simulink model "Combined_Experiment_Jan23_2020a"  (R2020a)
settings: Solver=FixedStepAuto  StartTime=0.0  StopTime=tsim  FixedStep=baseRate  RelTol=1e-3  EnableMultiTasking=on
undefined symbols (not defined in the file): b0, b1, b_out, baseRate, CHASER_ABSOLUTE_POSITION, DiscIntNeverNeededParam, drop_states_ARM, drop_states_BLACK, drop_states_BLUE, drop_states_RED, F_Black_X_nominal, F_Black_Y_nominal, F_Blue_X_nominal, F_Blue_Y_nominal, F_red_X_nominal, F_red_Y_nominal, F_thrusters_BLACK, F_thrusters_BLUE, F_thrusters_RED, Gamma1_el, Gamma1_sh, Gamma1_wr, Gamma2_el, Gamma2_sh, Gamma2_wr, Gamma3_el, Gamma3_sh, Gamma3_wr, Gamma4_el, Gamma4_sh, Gamma4_wr, Gamma5_el, Gamma5_sh, Gamma5_wr, Gamma6_el, Gamma6_sh, Gamma6_wr, home_states_BLACK, home_states_BLUE, home_states_RED, init_states_BLACK, init_states_BLUE, init_states_RED, Kd_tb, Kd_tblue, Kd_tr, Kd_xb, Kd_xblue, Kd_xr, Kd_yb, Kd_yblue, Kd_yr, Kp_tb, Kp_tblue, Kp_tr, Kp_xb, Kp_xblue, Kp_xr, Kp_yb, Kp_yblue ... (+31)
libraries: dspstat3 x18, raspberrypiBasiclib x10, dspsigops x9, embdlinuxlib x8, MainLibrary x8, simulink x7, mspfiltlib x3, dsparch4 x3, etargetslib x1, sensehatlib x1
(part 5 of 11)

== system Combined_Experiment_Jan23_2020a/Phase #3: Experiment/Change BLUE Behavior/Sub-Phase #3  ==
  note: Additional blocks are stored here.
  note: A simple PD control law is used here to command the platform to it's initial position, as defined in the initializer.
  note: Additional Blocks
  note: PD Control Law - BLUE
  Action Port : ActionPort  ActionPortLabel=elseif( u1 < u4)
  BLACK_Rz : DataStoreRead  DataStoreName=BLUE_Rz
  BLACK_RzD1 : Subsystem
  BLACK_Tz : DataStoreWrite  DataStoreName=BLUE_Tz
  BLUE_Fx : DataStoreWrite  DataStoreName=BLUE_Fx
  BLUE_Fy : DataStoreWrite  DataStoreName=BLUE_Fy
  BLUE_Px : DataStoreRead  DataStoreName=BLUE_Px
  "BLUE_Py " : DataStoreRead  DataStoreName=BLUE_Py
  Constant : Constant  Value=xLength/2
  Constant1 : Constant  Value=yLength/2
  Custom Discrete PD (Attitude) : Subsystem
  Custom Discrete PD (X-Position) : Subsystem
  Custom Discrete PD (Y-Position) : Subsystem
  Data Store Write1 : DataStoreWrite  DataStoreName=Float_State
  Hough Control : Subsystem
  Puck State : Constant
  Subtract : Sum  Inputs=+-
  Subtract1 : Sum  Inputs=+-
  wires:
  Puck State/1 -> Data Store Write1/1
  BLACK_RzD1/1(Ref) -> Hough Control/1(Ref)
  BLACK_Rz/1 -> Hough Control/2(Act)
  BLUE_Px/1 -> Subtract/2
  "BLUE_Py "/1 -> Subtract1/2
  Subtract1/1 -> Custom Discrete PD (Y-Position)/1(ey)
  Subtract/1 -> Custom Discrete PD (X-Position)/1(ex)
  Custom Discrete PD (Y-Position)/1(Fy) -> BLUE_Fy/1
  Hough Control/1(Err) -> Custom Discrete PD (Attitude)/1(ez)
  Custom Discrete PD (Attitude)/1(Tz) -> BLACK_Tz/1
  Custom Discrete PD (X-Position)/1(Fx) -> BLUE_Fx/1
  Constant1/1 -> Subtract1/1
  Constant/1 -> Subtract/1

== system Combined_Experiment_Jan23_2020a/Phase #3: Experiment/Change BLUE Behavior/Sub-Phase #4 ==
  note: Additional blocks are stored here.
  note: A simple PD control law is used here to command the platform to it's initial position, as defined in the initializer.
  note: Additional Blocks
  note: PD Control Law - BLUE
  Action Port : ActionPort  ActionPortLabel=elseif( u1 < u5)
  BLACK_Rz : DataStoreRead  DataStoreName=BLUE_Rz
  BLACK_RzD1 : Subsystem
  BLACK_Tz : DataStoreWrite  DataStoreName=BLUE_Tz
  BLUE_Fx : DataStoreWrite  DataStoreName=BLUE_Fx
  BLUE_Fy : DataStoreWrite  DataStoreName=BLUE_Fy
  BLUE_Px : DataStoreRead  DataStoreName=BLUE_Px
  "BLUE_Py " : DataStoreRead  DataStoreName=BLUE_Py
  Constant : Constant  Value=xLength/2
  Constant1 : Constant  Value=yLength/2
  Custom Discrete PD (Attitude) : Subsystem
  Custom Discrete PD (X-Position) : Subsystem
  Custom Discrete PD (Y-Position) : Subsystem
  Data Store Write1 : DataStoreWrite  DataStoreName=Float_State
  Hough Control : Subsystem
  Puck State : Constant
  Subtract : Sum  Inputs=+-
  Subtract1 : Sum  Inputs=+-
  wires:
  Puck State/1 -> Data Store Write1/1
  BLACK_RzD1/1(Ref) -> Hough Control/1(Ref)
  BLACK_Rz/1 -> Hough Control/2(Act)
  BLUE_Px/1 -> Subtract/2
  "BLUE_Py "/1 -> Subtract1/2
  Subtract1/1 -> Custom Discrete PD (Y-Position)/1(ey)
  Subtract/1 -> Custom Discrete PD (X-Position)/1(ex)
  Custom Discrete PD (Y-Position)/1(Fy) -> BLUE_Fy/1
  Hough Control/1(Err) -> Custom Discrete PD (Attitude)/1(ez)
  Custom Discrete PD (Attitude)/1(Tz) -> BLACK_Tz/1
  Custom Discrete PD (X-Position)/1(Fx) -> BLUE_Fx/1
  Constant1/1 -> Subtract1/1
  Constant/1 -> Subtract/1

== system Combined_Experiment_Jan23_2020a/Phase #3: Experiment/Change BLUE Behavior/Subsystem ==
  Universal_Time : DataStoreRead  DataStoreName=Univ_Time
  Time : Outport  VectorParamsAs1DForOutWhenUnconnected=off
  wires:
  Universal_Time/1 -> Time/1

== system Combined_Experiment_Jan23_2020a/Phase #3: Experiment/Change RED Behavior/Sub-Phase #1 ==
  note: Additional Blocks
  note: Additional blocks are stored above. Note that to control attitude using the RW, simply replace RED_Tz with RED_Tz_RW.
  note: Feedforward control
  note: ARM Control Law - RED
  Action Port : ActionPort  ActionPortLabel=if(u1 < u2)
  Constant1 : Constant  Value=0
  Constant4 : Constant  Value=platformSelection
  Data Store Write3 : DataStoreWrite  DataStoreName=Float_State
  Demux1 : Demux  Outputs=3
  If : If  IfExpression=u1 == 4 | u1 == 5 | u1 == 10 | u1 == 11
  Mux3 : Mux  Inputs=3
  Product : Product  Multiplication=Matrix(*)
  Puck State : Constant
  RED : Subsystem  TreatAsAtomicUnit=on
  RED+ARM : Subsystem  TreatAsAtomicUnit=on
  RED_Desired_Ax : DataStoreRead  DataStoreName=RED_Desired_Ax
  RED_Desired_Ay : DataStoreRead  DataStoreName=RED_Desired_Ay
  RED_Desired_Omega : DataStoreRead  DataStoreName=RED_Desired_Alpha
  RED_Fx : DataStoreWrite  DataStoreName=RED_Fx
  RED_Fy : DataStoreWrite  DataStoreName=RED_Fy
  RED_Tz : DataStoreWrite  DataStoreName=RED_Tz
  RED_Tz_RW : DataStoreWrite  DataStoreName=RED_Tz_RW
  calculate_mass_matrix : MATLAB Function  TreatAsAtomicUnit=on
  wires:
  Constant1/1 -> RED_Tz_RW/1
  Puck State/1 -> Data Store Write3/1
  Product/1 -> Demux1/1
  RED_Desired_Omega/1 -> Mux3/3
  RED_Desired_Ay/1 -> Mux3/2
  calculate_mass_matrix/1(M) -> Product/1
  RED_Desired_Ax/1 -> Mux3/1
  Mux3/1 -> Product/2
  Demux1/1 -> RED_Fx/1
  Demux1/2 -> RED_Fy/1
  Demux1/3 -> RED_Tz/1
  If/1 -> RED+ARM/Action
  If/2 -> RED/Action
  Constant4/1 -> If/1

== system Combined_Experiment_Jan23_2020a/Phase #3: Experiment/Change RED Behavior/Sub-Phase #2  ==
  note: Feedforward control
  note: Additional Blocks
  note: ARM Control Law - RED
  note: Additional blocks are stored above. Note that to control attitude using the RW, simply replace RED_Tz with RED_Tz_RW.
  Action Port : ActionPort  ActionPortLabel=elseif(u1 < u3)
  Constant1 : Constant  Value=0
  Constant4 : Constant  Value=platformSelection
  Data Store Write3 : DataStoreWrite  DataStoreName=Float_State
  Demux1 : Demux  Outputs=3
  If : If  IfExpression=u1 == 4 | u1 == 5 | u1 == 10 | u1 == 11
  Mux3 : Mux  Inputs=3
  Product : Product  Multiplication=Matrix(*)
  Puck State : Constant
  RED : Subsystem  TreatAsAtomicUnit=on
  RED+ARM : Subsystem  TreatAsAtomicUnit=on
  RED_Desired_Ax : DataStoreRead  DataStoreName=RED_Desired_Ax
  RED_Desired_Ay : DataStoreRead  DataStoreName=RED_Desired_Ay
  RED_Desired_Omega : DataStoreRead  DataStoreName=RED_Desired_Alpha
  RED_Fx : DataStoreWrite  DataStoreName=RED_Fx
  RED_Fy : DataStoreWrite  DataStoreName=RED_Fy
  RED_Tz : DataStoreWrite  DataStoreName=RED_Tz
  RED_Tz_RW : DataStoreWrite  DataStoreName=RED_Tz_RW
  calculate_mass_matrix : MATLAB Function  TreatAsAtomicUnit=on
  wires:
  Demux1/1 -> RED_Fx/1
  Mux3/1 -> Product/2
  Demux1/3 -> RED_Tz/1
  calculate_mass_matrix/1(M) -> Product/1
  Product/1 -> Demux1/1
  Demux1/2 -> RED_Fy/1
  Constant1/1 -> RED_Tz_RW/1
  RED_Desired_Omega/1 -> Mux3/3
  Puck State/1 -> Data Store Write3/1
  Constant4/1 -> If/1
  If/2 -> RED/Action
  RED_Desired_Ay/1 -> Mux3/2
  If/1 -> RED+ARM/Action
  RED_Desired_Ax/1 -> Mux3/1

== system Combined_Experiment_Jan23_2020a/Phase #3: Experiment/Change RED Behavior/Sub-Phase #3  ==
  note: Feedforward control
  note: Additional Blocks
  note: ARM Control Law - RED
  note: Additional blocks are stored above. Note that to control attitude using the RW, simply replace RED_Tz with RED_Tz_RW.
  Action Port : ActionPort  ActionPortLabel=elseif( u1 < u4)
  Constant1 : Constant  Value=0
  Constant4 : Constant  Value=platformSelection
  Data Store Write3 : DataStoreWrite  DataStoreName=Float_State
  Demux1 : Demux  Outputs=3
  If : If  IfExpression=u1 == 4 | u1 == 5 | u1 == 10 | u1 == 11
  Mux3 : Mux  Inputs=3
  Product : Product  Multiplication=Matrix(*)
  Puck State : Constant
  RED : Subsystem  TreatAsAtomicUnit=on
  RED+ARM : Subsystem  TreatAsAtomicUnit=on
  RED_Desired_Ax : DataStoreRead  DataStoreName=RED_Desired_Ax
  RED_Desired_Ay : DataStoreRead  DataStoreName=RED_Desired_Ay
  RED_Desired_Omega : DataStoreRead  DataStoreName=RED_Desired_Alpha
  RED_Fx : DataStoreWrite  DataStoreName=RED_Fx
  RED_Fy : DataStoreWrite  DataStoreName=RED_Fy
  RED_Tz : DataStoreWrite  DataStoreName=RED_Tz
  RED_Tz_RW : DataStoreWrite  DataStoreName=RED_Tz_RW
  calculate_mass_matrix : MATLAB Function  TreatAsAtomicUnit=on
  wires:
  Demux1/1 -> RED_Fx/1
  Mux3/1 -> Product/2
  calculate_mass_matrix/1(M) -> Product/1
  Product/1 -> Demux1/1
  Demux1/2 -> RED_Fy/1
  Constant1/1 -> RED_Tz_RW/1
  RED_Desired_Omega/1 -> Mux3/3
  Puck State/1 -> Data Store Write3/1
  Constant4/1 -> If/1
  If/2 -> RED/Action
  RED_Desired_Ay/1 -> Mux3/2
  If/1 -> RED+ARM/Action
  RED_Desired_Ax/1 -> Mux3/1
  Demux1/3 -> RED_Tz/1

== system Combined_Experiment_Jan23_2020a/Phase #3: Experiment/Change RED Behavior/Sub-Phase #4 ==
  note: Feedforward control
  note: Additional Blocks
  note: ARM Control Law - RED
  note: Additional blocks are stored above. Note that to control attitude using the RW, simply replace RED_Tz with RED_Tz_RW.
  Action Port : ActionPort  ActionPortLabel=elseif( u1 < u5)
  Constant1 : Constant  Value=0
  Constant4 : Constant  Value=platformSelection
  Data Store Write3 : DataStoreWrite  DataStoreName=Float_State
  Demux1 : Demux  Outputs=3
  If : If  IfExpression=u1 == 4 | u1 == 5 | u1 == 10 | u1 == 11
  Mux3 : Mux  Inputs=3
  Product : Product  Multiplication=Matrix(*)
  Puck State : Constant
  RED : Subsystem  TreatAsAtomicUnit=on
  RED+ARM : Subsystem  TreatAsAtomicUnit=on
  RED_Desired_Ax : DataStoreRead  DataStoreName=RED_Desired_Ax
  RED_Desired_Ay : DataStoreRead  DataStoreName=RED_Desired_Ay
  RED_Desired_Omega : DataStoreRead  DataStoreName=RED_Desired_Alpha
  RED_Fx : DataStoreWrite  DataStoreName=RED_Fx
  RED_Fy : DataStoreWrite  DataStoreName=RED_Fy
  RED_Tz : DataStoreWrite  DataStoreName=RED_Tz
  RED_Tz_RW : DataStoreWrite  DataStoreName=RED_Tz_RW
  calculate_mass_matrix : MATLAB Function  TreatAsAtomicUnit=on
  wires:
  Demux1/1 -> RED_Fx/1
  Mux3/1 -> Product/2
  Demux1/3 -> RED_Tz/1
  calculate_mass_matrix/1(M) -> Product/1
  Product/1 -> Demux1/1
  Demux1/2 -> RED_Fy/1
  Constant1/1 -> RED_Tz_RW/1
  RED_Desired_Omega/1 -> Mux3/3
  Puck State/1 -> Data Store Write3/1
  Constant4/1 -> If/1
  If/2 -> RED/Action
  RED_Desired_Ay/1 -> Mux3/2
  If/1 -> RED+ARM/Action
  RED_Desired_Ax/1 -> Mux3/1

== system Combined_Experiment_Jan23_2020a/Phase #3: Experiment/Change RED Behavior/Subsystem ==
  Universal_Time : DataStoreRead  DataStoreName=Univ_Time
  Time : Outport  VectorParamsAs1DForOutWhenUnconnected=off
  wires:
  Universal_Time/1 -> Time/1

== system Combined_Experiment_Jan23_2020a/Phase #4: Return Home/Change BLACK Behavior/Custom Discrete PD (Attitude) ==
  ez : Inport
  Sum3 : Sum
  kd_tb : Gain  Gain=Kd_tb
  kp_tb : Gain  Gain=Kp_tb
  "x_dot -> x1" : Subsystem
  Tz : Outport  VectorParamsAs1DForOutWhenUnconnected=off
  wires:
  kd_tb/1 -> Sum3/1
  Sum3/1 -> Tz/1
  kp_tb/1 -> Sum3/2
  "x_dot -> x1"/1(dy(t)/dt) -> kd_tb/1
  ez/1 -> "x_dot -> x1"/1(y(t)), kp_tb/1

== system Combined_Experiment_Jan23_2020a/Phase #4: Return Home/Change BLACK Behavior/Custom Discrete PD (X-Position) ==
  ex : Inport
  Sum3 : Sum
  kd_xb : Gain  Gain=Kd_xb
  kp_xb : Gain  Gain=Kp_xb
  "x_dot -> x1" : Subsystem
  Fx : Outport  VectorParamsAs1DForOutWhenUnconnected=off
  wires:
  kd_xb/1 -> Sum3/1
  ex/1 -> "x_dot -> x1"/1(y(t)), kp_xb/1
  kp_xb/1 -> Sum3/2
  "x_dot -> x1"/1(dy(t)/dt) -> kd_xb/1
  Sum3/1 -> Fx/1

== system Combined_Experiment_Jan23_2020a/Phase #4: Return Home/Change BLACK Behavior/Custom Discrete PD (Y-Position) ==
  ey : Inport
  Sum3 : Sum
  kd_yb : Gain  Gain=Kd_yb
  kp_yb : Gain  Gain=Kp_yb
  "x_dot -> x1" : Subsystem
  Fy : Outport  VectorParamsAs1DForOutWhenUnconnected=off
  wires:
  kd_yb/1 -> Sum3/1
  Sum3/1 -> Fy/1
  kp_yb/1 -> Sum3/2
  "x_dot -> x1"/1(dy(t)/dt) -> kd_yb/1
  ey/1 -> "x_dot -> x1"/1(y(t)), kp_yb/1

== system Combined_Experiment_Jan23_2020a/Phase #4: Return Home/Change BLACK Behavior/Hough Control ==
  Ref : Inport
  Act : Inport  Port=2
  MATLAB Function2 : MATLAB Function  TreatAsAtomicUnit=on
  MATLAB Function3 : MATLAB Function  TreatAsAtomicUnit=on
  MATLAB Function4 : MATLAB Function  TreatAsAtomicUnit=on
  Subtract2 : Sum  Inputs=+-
  Err : Outport  VectorParamsAs1DForOutWhenUnconnected=off
  wires:
  MATLAB Function4/1(e_out) -> Err/1
  MATLAB Function2/1(Oy) -> MATLAB Function4/1(Oy)
  Subtract2/1 -> MATLAB Function4/2(e_in)
  MATLAB Function2/2(Ox) -> Subtract2/1
  Act/1 -> MATLAB Function3/1(z)
  Ref/1 -> MATLAB Function2/1(z)
  MATLAB Function3/1(Ox) -> Subtract2/2

== system Combined_Experiment_Jan23_2020a/Phase #4: Return Home/Change BLUE Behavior/Custom Discrete PD (Attitude) ==
  ez : Inport
  Sum3 : Sum
  kd_tb : Gain  Gain=Kd_tblue
  kp_tb : Gain  Gain=Kp_tblue
  "x_dot -> x1" : Subsystem
  Tz : Outport  VectorParamsAs1DForOutWhenUnconnected=off
  wires:
  kd_tb/1 -> Sum3/1
  Sum3/1 -> Tz/1
  kp_tb/1 -> Sum3/2
  "x_dot -> x1"/1(dy(t)/dt) -> kd_tb/1
  ez/1 -> "x_dot -> x1"/1(y(t)), kp_tb/1

== system Combined_Experiment_Jan23_2020a/Phase #4: Return Home/Change BLUE Behavior/Custom Discrete PD (X-Position) ==
  ex : Inport
  Sum3 : Sum
  kd_xb : Gain  Gain=Kd_xblue
  kp_xb : Gain  Gain=Kp_xblue
  "x_dot -> x1" : Subsystem
  Fx : Outport  VectorParamsAs1DForOutWhenUnconnected=off
  wires:
  kd_xb/1 -> Sum3/1
  ex/1 -> "x_dot -> x1"/1(y(t)), kp_xb/1
  kp_xb/1 -> Sum3/2
  "x_dot -> x1"/1(dy(t)/dt) -> kd_xb/1
  Sum3/1 -> Fx/1

== system Combined_Experiment_Jan23_2020a/Phase #4: Return Home/Change BLUE Behavior/Custom Discrete PD (Y-Position) ==
  ey : Inport
  Sum3 : Sum
  kd_yb : Gain  Gain=Kd_yblue
  kp_yb : Gain  Gain=Kp_yblue
  "x_dot -> x1" : Subsystem
  Fy : Outport  VectorParamsAs1DForOutWhenUnconnected=off
  wires:
  kd_yb/1 -> Sum3/1
  Sum3/1 -> Fy/1
  kp_yb/1 -> Sum3/2
  "x_dot -> x1"/1(dy(t)/dt) -> kd_yb/1
  ey/1 -> "x_dot -> x1"/1(y(t)), kp_yb/1

== system Combined_Experiment_Jan23_2020a/Phase #4: Return Home/Change BLUE Behavior/Hough Control ==
  Ref : Inport
  Act : Inport  Port=2
  MATLAB Function2 : MATLAB Function  TreatAsAtomicUnit=on
  MATLAB Function3 : MATLAB Function  TreatAsAtomicUnit=on
  MATLAB Function4 : MATLAB Function  TreatAsAtomicUnit=on
  Subtract2 : Sum  Inputs=+-
  Err : Outport  VectorParamsAs1DForOutWhenUnconnected=off
  wires:
  MATLAB Function4/1(e_out) -> Err/1
  MATLAB Function2/1(Oy) -> MATLAB Function4/1(Oy)
  Subtract2/1 -> MATLAB Function4/2(e_in)
  MATLAB Function2/2(Ox) -> Subtract2/1
  Act/1 -> MATLAB Function3/1(z)
  Ref/1 -> MATLAB Function2/1(z)
  MATLAB Function3/1(Ox) -> Subtract2/2

== system Combined_Experiment_Jan23_2020a/Phase #4: Return Home/Change RED Behavior/Custom Discrete PD (Attitude) ==
  ez : Inport
  Sum3 : Sum
  kd_tr : Gain  Gain=Kd_tr
  kp_tr : Gain  Gain=Kp_tr
  "x_dot -> x2" : Subsystem
  Tz : Outport  VectorParamsAs1DForOutWhenUnconnected=off
  wires:
  kd_tr/1 -> Sum3/1
  Sum3/1 -> Tz/1
  kp_tr/1 -> Sum3/2
  "x_dot -> x2"/1(dy(t)/dt) -> kd_tr/1
  ez/1 -> "x_dot -> x2"/1(y(t)), kp_tr/1

== system Combined_Experiment_Jan23_2020a/Phase #4: Return Home/Change RED Behavior/Custom Discrete PD (X-Position) ==
  ex : Inport
  Sum3 : Sum
  kd_xr : Gain  Gain=Kd_xr
  kp_xr : Gain  Gain=Kp_xr
  "x_dot -> x2" : Subsystem
  Fx : Outport  VectorParamsAs1DForOutWhenUnconnected=off
  wires:
  kd_xr/1 -> Sum3/1
  ex/1 -> "x_dot -> x2"/1(y(t)), kp_xr/1
  kp_xr/1 -> Sum3/2
  "x_dot -> x2"/1(dy(t)/dt) -> kd_xr/1
  Sum3/1 -> Fx/1

== system Combined_Experiment_Jan23_2020a/Phase #4: Return Home/Change RED Behavior/Custom Discrete PD (Y-Position) ==
  ey : Inport
  Sum3 : Sum
  kd_yr : Gain  Gain=Kd_yr
  kp_yr : Gain  Gain=Kp_yr
  "x_dot -> x2" : Subsystem
  Fy : Outport  VectorParamsAs1DForOutWhenUnconnected=off
  wires:
  kd_yr/1 -> Sum3/1
  Sum3/1 -> Fy/1
  kp_yr/1 -> Sum3/2
  "x_dot -> x2"/1(dy(t)/dt) -> kd_yr/1
  ey/1 -> "x_dot -> x2"/1(y(t)), kp_yr/1

== system Combined_Experiment_Jan23_2020a/Phase #4: Return Home/Change RED Behavior/Hough Control ==
  Ref : Inport
  Act : Inport  Port=2
  MATLAB Function2 : MATLAB Function  TreatAsAtomicUnit=on
  MATLAB Function3 : MATLAB Function  TreatAsAtomicUnit=on
  MATLAB Function4 : MATLAB Function  TreatAsAtomicUnit=on
  Subtract2 : Sum  Inputs=+-
  Err : Outport  VectorParamsAs1DForOutWhenUnconnected=off
  wires:
  MATLAB Function4/1(e_out) -> Err/1
  MATLAB Function2/1(Oy) -> MATLAB Function4/1(Oy)
  Subtract2/1 -> MATLAB Function4/2(e_in)
  MATLAB Function2/2(Ox) -> Subtract2/1
  Act/1 -> MATLAB Function3/1(z)
  Ref/1 -> MATLAB Function2/1(z)
  MATLAB Function3/1(Ox) -> Subtract2/2

== system Combined_Experiment_Jan23_2020a/Phase #4: Return Home/Change RED Behavior/RED ==
  note: ARM Control Law - RED
  note: When the ARM is not in use, send zeros.
  Action Port : ActionPort  ActionPortLabel=else
  ARM_Desired_Rz_Elbow : DataStoreWrite  Commented=on  DataStoreName=ARM_Desired_Rz_Elbow
  ARM_Desired_Rz_Shoulder : DataStoreWrite  Commented=on  DataStoreName=ARM_Desired_Rz_Shoulder
  ARM_Desired_Rz_Wrist : DataStoreWrite  Commented=on  DataStoreName=ARM_Desired_Rz_Wrist
  Constant1 : Constant  Commented=on  Value=pi/2
  Constant7 : Constant  Commented=on  Value=0
  wires:
  Constant7/1 -> ARM_Desired_Rz_Wrist/1
  Constant1/1 -> ARM_Desired_Rz_Shoulder/1, ARM_Desired_Rz_Elbow/1

== system Combined_Experiment_Jan23_2020a/Phase #4: Return Home/Change RED Behavior/RED+ARM ==
  note: ARM Control Law - RED
  note: This section is reserved for any control law for the robotic manipulator.
  Action Port : ActionPort  ActionPortLabel=if(u1 == 4 | u1 == 5 | u1 == 10 | u1 == 11)
  ARM_Desired_Rz_Elbow : DataStoreWrite  Commented=on  DataStoreName=ARM_Desired_Rz_Elbow
  ARM_Desired_Rz_Elbow1 : DataStoreWrite  DataStoreName=ARM_Desired_Rz_Elbow
  ARM_Desired_Rz_Shoulder : DataStoreWrite  Commented=on  DataStoreName=ARM_Desired_Rz_Shoulder
  ARM_Desired_Rz_Shoulder1 : DataStoreWrite  DataStoreName=ARM_Desired_Rz_Shoulder
  ARM_Desired_Rz_Wrist : DataStoreWrite  Commented=on  DataStoreName=ARM_Desired_Rz_Wrist
  ARM_Desired_Rz_Wrist1 : DataStoreWrite  DataStoreName=ARM_Desired_Rz_Wrist
  Constant : Constant  Value=-1.415
  Constant1 : Constant  Commented=on  Value=pi/2
  Constant2 : Constant  Value=-1.13000000000000
  Constant3 : Constant  Value=0.98
  Constant7 : Constant  Commented=on  Value=0
  wires:
  Constant7/1 -> ARM_Desired_Rz_Wrist/1
  Constant1/1 -> ARM_Desired_Rz_Shoulder/1, ARM_Desired_Rz_Elbow/1
  Constant2/1 -> ARM_Desired_Rz_Shoulder1/1
  Constant/1 -> ARM_Desired_Rz_Elbow1/1
  Constant3/1 -> ARM_Desired_Rz_Wrist1/1

== system Combined_Experiment_Jan23_2020a/Phase #5: Hold Home/Change BLACK Behavior/Custom Discrete PD (Attitude) ==
  ez : Inport
  Sum3 : Sum
  kd_tb : Gain  Gain=Kd_tb
  kp_tb : Gain  Gain=Kp_tb
  "x_dot -> x1" : Subsystem
  Tz : Outport  VectorParamsAs1DForOutWhenUnconnected=off
  wires:
  kd_tb/1 -> Sum3/1
  Sum3/1 -> Tz/1
  kp_tb/1 -> Sum3/2
  "x_dot -> x1"/1(dy(t)/dt) -> kd_tb/1
  ez/1 -> "x_dot -> x1"/1(y(t)), kp_tb/1

== system Combined_Experiment_Jan23_2020a/Phase #5: Hold Home/Change BLACK Behavior/Custom Discrete PD (X-Position) ==
  ex : Inport
  Sum3 : Sum
  kd_xb : Gain  Gain=Kd_xb
  kp_xb : Gain  Gain=Kp_xb
  "x_dot -> x1" : Subsystem
  Fx : Outport  VectorParamsAs1DForOutWhenUnconnected=off
  wires:
  kd_xb/1 -> Sum3/1
  ex/1 -> "x_dot -> x1"/1(y(t)), kp_xb/1
  kp_xb/1 -> Sum3/2
  "x_dot -> x1"/1(dy(t)/dt) -> kd_xb/1
  Sum3/1 -> Fx/1

== system Combined_Experiment_Jan23_2020a/Phase #5: Hold Home/Change BLACK Behavior/Custom Discrete PD (Y-Position) ==
  ey : Inport
  Sum3 : Sum
  kd_yb : Gain  Gain=Kd_yb
  kp_yb : Gain  Gain=Kp_yb
  "x_dot -> x1" : Subsystem
  Fy : Outport  VectorParamsAs1DForOutWhenUnconnected=off
  wires:
  kd_yb/1 -> Sum3/1
  Sum3/1 -> Fy/1
  kp_yb/1 -> Sum3/2
  "x_dot -> x1"/1(dy(t)/dt) -> kd_yb/1
  ey/1 -> "x_dot -> x1"/1(y(t)), kp_yb/1

== system Combined_Experiment_Jan23_2020a/Phase #5: Hold Home/Change BLACK Behavior/Hough Control ==
  Ref : Inport
  Act : Inport  Port=2
  MATLAB Function2 : MATLAB Function  TreatAsAtomicUnit=on
  MATLAB Function3 : MATLAB Function  TreatAsAtomicUnit=on
  MATLAB Function4 : MATLAB Function  TreatAsAtomicUnit=on
  Subtract2 : Sum  Inputs=+-
  Err : Outport  VectorParamsAs1DForOutWhenUnconnected=off
  wires:
  MATLAB Function4/1(e_out) -> Err/1
  MATLAB Function2/1(Oy) -> MATLAB Function4/1(Oy)
  Subtract2/1 -> MATLAB Function4/2(e_in)
  MATLAB Function2/2(Ox) -> Subtract2/1
  Act/1 -> MATLAB Function3/1(z)
  Ref/1 -> MATLAB Function2/1(z)
  MATLAB Function3/1(Ox) -> Subtract2/2

== system Combined_Experiment_Jan23_2020a/Phase #5: Hold Home/Change BLUE Behavior/Custom Discrete PD (Attitude) ==
  ez : Inport
  Sum3 : Sum
  kd_tb : Gain  Gain=Kd_tblue
  kp_tb : Gain  Gain=Kp_tblue
  "x_dot -> x1" : Subsystem
  Tz : Outport  VectorParamsAs1DForOutWhenUnconnected=off
  wires:
  kd_tb/1 -> Sum3/1
  Sum3/1 -> Tz/1
  kp_tb/1 -> Sum3/2
  "x_dot -> x1"/1(dy(t)/dt) -> kd_tb/1
  ez/1 -> "x_dot -> x1"/1(y(t)), kp_tb/1

== system Combined_Experiment_Jan23_2020a/Phase #5: Hold Home/Change BLUE Behavior/Custom Discrete PD (X-Position) ==
  ex : Inport
  Sum3 : Sum
  kd_xb : Gain  Gain=Kd_xblue
  kp_xb : Gain  Gain=Kp_xblue
  "x_dot -> x1" : Subsystem
  Fx : Outport  VectorParamsAs1DForOutWhenUnconnected=off
  wires:
  kd_xb/1 -> Sum3/1
  ex/1 -> "x_dot -> x1"/1(y(t)), kp_xb/1
  kp_xb/1 -> Sum3/2
  "x_dot -> x1"/1(dy(t)/dt) -> kd_xb/1
  Sum3/1 -> Fx/1

== system Combined_Experiment_Jan23_2020a/Phase #5: Hold Home/Change BLUE Behavior/Custom Discrete PD (Y-Position) ==
  ey : Inport
  Sum3 : Sum
  kd_yb : Gain  Gain=Kd_yblue
  kp_yb : Gain  Gain=Kp_yblue
  "x_dot -> x1" : Subsystem
  Fy : Outport  VectorParamsAs1DForOutWhenUnconnected=off
  wires:
  kd_yb/1 -> Sum3/1
  Sum3/1 -> Fy/1
  kp_yb/1 -> Sum3/2
  "x_dot -> x1"/1(dy(t)/dt) -> kd_yb/1
  ey/1 -> "x_dot -> x1"/1(y(t)), kp_yb/1

== system Combined_Experiment_Jan23_2020a/Phase #5: Hold Home/Change BLUE Behavior/Hough Control ==
  Ref : Inport
  Act : Inport  Port=2
  MATLAB Function2 : MATLAB Function  TreatAsAtomicUnit=on
  MATLAB Function3 : MATLAB Function  TreatAsAtomicUnit=on
  MATLAB Function4 : MATLAB Function  TreatAsAtomicUnit=on
  Subtract2 : Sum  Inputs=+-
  Err : Outport  VectorParamsAs1DForOutWhenUnconnected=off
  wires:
  MATLAB Function4/1(e_out) -> Err/1
  MATLAB Function2/1(Oy) -> MATLAB Function4/1(Oy)
  Subtract2/1 -> MATLAB Function4/2(e_in)
  MATLAB Function2/2(Ox) -> Subtract2/1
  Act/1 -> MATLAB Function3/1(z)
  Ref/1 -> MATLAB Function2/1(z)
  MATLAB Function3/1(Ox) -> Subtract2/2

== system Combined_Experiment_Jan23_2020a/Phase #5: Hold Home/Change RED Behavior/Custom Discrete PD (Attitude) ==
  ez : Inport
  Sum3 : Sum
  kd_tr : Gain  Gain=Kd_tr
  kp_tr : Gain  Gain=Kp_tr
  "x_dot -> x2" : Subsystem
  Tz : Outport  VectorParamsAs1DForOutWhenUnconnected=off
  wires:
  kd_tr/1 -> Sum3/1
  Sum3/1 -> Tz/1
  kp_tr/1 -> Sum3/2
  "x_dot -> x2"/1(dy(t)/dt) -> kd_tr/1
  ez/1 -> "x_dot -> x2"/1(y(t)), kp_tr/1

== system Combined_Experiment_Jan23_2020a/Phase #5: Hold Home/Change RED Behavior/Custom Discrete PD (X-Position) ==
  ex : Inport
  Sum3 : Sum
  kd_xr : Gain  Gain=Kd_xr
  kp_xr : Gain  Gain=Kp_xr
  "x_dot -> x2" : Subsystem
  Fx : Outport  VectorParamsAs1DForOutWhenUnconnected=off
  wires:
  kd_xr/1 -> Sum3/1
  ex/1 -> "x_dot -> x2"/1(y(t)), kp_xr/1
  kp_xr/1 -> Sum3/2
  "x_dot -> x2"/1(dy(t)/dt) -> kd_xr/1
  Sum3/1 -> Fx/1

== system Combined_Experiment_Jan23_2020a/Phase #5: Hold Home/Change RED Behavior/Custom Discrete PD (Y-Position) ==
  ey : Inport
  Sum3 : Sum
  kd_yr : Gain  Gain=Kd_yr
  kp_yr : Gain  Gain=Kp_yr
  "x_dot -> x2" : Subsystem
  Fy : Outport  VectorParamsAs1DForOutWhenUnconnected=off
  wires:
  kd_yr/1 -> Sum3/1
  Sum3/1 -> Fy/1
  kp_yr/1 -> Sum3/2
  "x_dot -> x2"/1(dy(t)/dt) -> kd_yr/1
  ey/1 -> "x_dot -> x2"/1(y(t)), kp_yr/1

== system Combined_Experiment_Jan23_2020a/Phase #5: Hold Home/Change RED Behavior/Hough Control ==
  Ref : Inport
  Act : Inport  Port=2
  MATLAB Function2 : MATLAB Function  TreatAsAtomicUnit=on
  MATLAB Function3 : MATLAB Function  TreatAsAtomicUnit=on
  MATLAB Function4 : MATLAB Function  TreatAsAtomicUnit=on
  Subtract2 : Sum  Inputs=+-
  Err : Outport  VectorParamsAs1DForOutWhenUnconnected=off
  wires:
  MATLAB Function4/1(e_out) -> Err/1
  MATLAB Function2/1(Oy) -> MATLAB Function4/1(Oy)
  Subtract2/1 -> MATLAB Function4/2(e_in)
  MATLAB Function2/2(Ox) -> Subtract2/1
  Act/1 -> MATLAB Function3/1(z)
  Ref/1 -> MATLAB Function2/1(z)
  MATLAB Function3/1(Ox) -> Subtract2/2

== system Combined_Experiment_Jan23_2020a/Phase #5: Hold Home/Change RED Behavior/RED ==
  note: ARM Control Law - RED
  note: When the ARM is not in use, send zeros.
  Action Port : ActionPort  ActionPortLabel=else
  ARM_Desired_Rz_Elbow : DataStoreWrite  Commented=on  DataStoreName=ARM_Desired_Rz_Elbow
  ARM_Desired_Rz_Shoulder : DataStoreWrite  Commented=on  DataStoreName=ARM_Desired_Rz_Shoulder
  ARM_Desired_Rz_Wrist : DataStoreWrite  Commented=on  DataStoreName=ARM_Desired_Rz_Wrist
  Constant1 : Constant  Commented=on  Value=pi/2
  Constant7 : Constant  Commented=on  Value=0
  wires:
  Constant7/1 -> ARM_Desired_Rz_Wrist/1
  Constant1/1 -> ARM_Desired_Rz_Shoulder/1, ARM_Desired_Rz_Elbow/1

== system Combined_Experiment_Jan23_2020a/Phase #5: Hold Home/Change RED Behavior/RED+ARM ==
  note: ARM Control Law - RED
  note: This section is reserved for any control law for the robotic manipulator.
  Action Port : ActionPort  ActionPortLabel=if(u1 == 4 | u1 == 5 | u1 == 10 | u1 == 11)
  ARM_Desired_Rz_Elbow : DataStoreWrite  Commented=on  DataStoreName=ARM_Desired_Rz_Elbow
  ARM_Desired_Rz_Elbow1 : DataStoreWrite  DataStoreName=ARM_Desired_Rz_Elbow
  ARM_Desired_Rz_Shoulder : DataStoreWrite  Commented=on  DataStoreName=ARM_Desired_Rz_Shoulder
  ARM_Desired_Rz_Shoulder1 : DataStoreWrite  DataStoreName=ARM_Desired_Rz_Shoulder
  ARM_Desired_Rz_Wrist : DataStoreWrite  Commented=on  DataStoreName=ARM_Desired_Rz_Wrist
  ARM_Desired_Rz_Wrist1 : DataStoreWrite  DataStoreName=ARM_Desired_Rz_Wrist
  Constant : Constant  Value=-1.415
  Constant1 : Constant  Commented=on  Value=pi/2
  Constant2 : Constant  Value=-1.13000000000000
  Constant3 : Constant  Value=0.98
  Constant7 : Constant  Commented=on  Value=0
  wires:
  Constant7/1 -> ARM_Desired_Rz_Wrist/1
  Constant1/1 -> ARM_Desired_Rz_Shoulder/1, ARM_Desired_Rz_Elbow/1
  Constant3/1 -> ARM_Desired_Rz_Wrist1/1
  Constant2/1 -> ARM_Desired_Rz_Shoulder1/1
  Constant/1 -> ARM_Desired_Rz_Elbow1/1

== system Combined_Experiment_Jan23_2020a/Simulate Plant Dynamics/BLACK Dynamics/BLACK Dynamics Model ==
  control_inputs : Inport
  Acceleration to Velocity : DiscreteIntegrator  IntegratorMethod=Integration: Backward Euler  SampleTime=-1  ICPrevOutput=DiscIntNeverNeededParam  ICPrevScaledInput=DiscIntNeverNeededParam
  MATLAB Function : MATLAB Function  TreatAsAtomicUnit=on
  Random Number : RandomNumber  Variance=noise_variance_BLACK
  Sum : Sum  Inputs=|++
  Velocity to Position : DiscreteIntegrator  IntegratorMethod=Integration: Backward Euler  InitialCondition=drop_states_BLACK  SampleTime=-1  ICPrevOutput=DiscIntNeverNeededParam  ICPrevScaledInput=DiscIntNeverNeededParam
  states : Outport  VectorParamsAs1DForOutWhenUnconnected=off
  wires:
  control_inputs/1 -> MATLAB Function/1(control_inputs)
  MATLAB Function/1(x_ddot) -> Acceleration to Velocity/1
  Acceleration to Velocity/1 -> Velocity to Position/1
  Velocity to Position/1 -> Sum/1
  Sum/1 -> states/1
  Random Number/1 -> Sum/2

== system Combined_Experiment_Jan23_2020a/Simulate Plant Dynamics/BLACK Dynamics/Sample and Hold Data to Match PhaseSpace (BLACK) ==
  states : Inport
  Constant1 : Constant  Value=serverRate
  Data Store Read2 : DataStoreRead  DataStoreName=Univ_Time
  MATLAB Function : MATLAB Function  TreatAsAtomicUnit=on
  Sample and Hold1 : dspsigops/Sample and Hold  trig=Rising edge  initCond=drop_states_BLACK  latchinput=off
  states_hold : Outport  VectorParamsAs1DForOutWhenUnconnected=off
  wires:
  states/1 -> Sample and Hold1/1
  Data Store Read2/1 -> MATLAB Function/1(TIME)
  Constant1/1 -> MATLAB Function/2(SERVER)
  MATLAB Function/1(y) -> Sample and Hold1/Trigger
  Sample and Hold1/1 -> states_hold/1

== system Combined_Experiment_Jan23_2020a/Simulate Plant Dynamics/BLACK Dynamics/x_dot -> x1 ==
  note: dy/dt ~= (y2-y1)/deltaT
  y(t) : Inport
  Delay1 : Delay  DelayLength=1  InitialConditionSource=Input port
      settings: InputPortMap=u0,p4
  Hold this value : Subsystem  TreatAsAtomicUnit=on
  Sum6 : Sum  Inputs=-+|
  divide by delta T : Gain  Gain=1/baseRate
  "if we went through a \"step\"" : If  IfExpression=u1 ~= 0  ShowElse=off
  dy(t)/dt : Outport  VectorParamsAs1DForOutWhenUnconnected=off
  wires:
  divide by delta T/1 -> dy(t)/dt/1
  Delay1/1 -> Sum6/1
  "if we went through a \"step\""/1 -> Hold this value/Action
  Hold this value/1(Out1) -> divide by delta T/1
  Sum6/1 -> "if we went through a \"step\""/1, Hold this value/1(In1)
  y(t)/1 -> Sum6/2, Delay1/2, Delay1/1

== system Combined_Experiment_Jan23_2020a/Simulate Plant Dynamics/BLACK Dynamics/x_dot -> x2 ==
  note: dy/dt ~= (y2-y1)/deltaT
  y(t) : Inport
  Delay1 : Delay  DelayLength=1  InitialConditionSource=Input port
      settings: InputPortMap=u0,p4
  Hold this value : Subsystem  TreatAsAtomicUnit=on
  Sum6 : Sum  Inputs=-+|
  divide by delta T : Gain  Gain=1/baseRate
  "if we went through a \"step\"" : If  IfExpression=u1 ~= 0  ShowElse=off
  dy(t)/dt : Outport  VectorParamsAs1DForOutWhenUnconnected=off
  wires:
  divide by delta T/1 -> dy(t)/dt/1
  Delay1/1 -> Sum6/1
  "if we went through a \"step\""/1 -> Hold this value/Action
  Hold this value/1(Out1) -> divide by delta T/1
  Sum6/1 -> "if we went through a \"step\""/1, Hold this value/1(In1)
  y(t)/1 -> Sum6/2, Delay1/2, Delay1/1

== system Combined_Experiment_Jan23_2020a/Simulate Plant Dynamics/BLACK Dynamics/x_dot -> x3 ==
  note: dy/dt ~= (y2-y1)/deltaT
  y(t) : Inport
  Delay1 : Delay  DelayLength=1  InitialConditionSource=Input port
      settings: InputPortMap=u0,p4
  Hold this value : Subsystem  TreatAsAtomicUnit=on
  Sum6 : Sum  Inputs=-+|
  divide by delta T : Gain  Gain=1/baseRate
  "if we went through a \"step\"" : If  IfExpression=u1 ~= 0  ShowElse=off
  dy(t)/dt : Outport  VectorParamsAs1DForOutWhenUnconnected=off
  wires:
  divide by delta T/1 -> dy(t)/dt/1
  Delay1/1 -> Sum6/1
  "if we went through a \"step\""/1 -> Hold this value/Action
  Hold this value/1(Out1) -> divide by delta T/1
  Sum6/1 -> "if we went through a \"step\""/1, Hold this value/1(In1)
  y(t)/1 -> Sum6/2, Delay1/2, Delay1/1

== system Combined_Experiment_Jan23_2020a/Simulate Plant Dynamics/BLACK Dynamics/x_dot -> x4 ==
  note: dy/dt ~= (y2-y1)/deltaT
  y(t) : Inport
  Delay1 : Delay  DelayLength=1  InitialConditionSource=Input port
      settings: InputPortMap=u0,p4
  Hold this value : Subsystem  TreatAsAtomicUnit=on
  Sum6 : Sum  Inputs=-+|
  divide by delta T : Gain  Gain=1/baseRate
  "if we went through a \"step\"" : If  IfExpression=u1 ~= 0  ShowElse=off
  dy(t)/dt : Outport  VectorParamsAs1DForOutWhenUnconnected=off
  wires:
  divide by delta T/1 -> dy(t)/dt/1
  Delay1/1 -> Sum6/1
  "if we went through a \"step\""/1 -> Hold this value/Action
  Hold this value/1(Out1) -> divide by delta T/1
  Sum6/1 -> "if we went through a \"step\""/1, Hold this value/1(In1)
  y(t)/1 -> Sum6/2, Delay1/2, Delay1/1

== system Combined_Experiment_Jan23_2020a/Simulate Plant Dynamics/BLACK Dynamics/x_dot -> x7 ==
  note: dy/dt ~= (y2-y1)/deltaT
  y(t) : Inport
  Delay1 : Delay  DelayLength=1  InitialConditionSource=Input port
      settings: InputPortMap=u0,p4
  Hold this value : Subsystem  TreatAsAtomicUnit=on
  Sum6 : Sum  Inputs=-+|
  divide by delta T : Gain  Gain=1/baseRate
  "if we went through a \"step\"" : If  IfExpression=u1 ~= 0  ShowElse=off
  dy(t)/dt : Outport  VectorParamsAs1DForOutWhenUnconnected=off
  wires:
  divide by delta T/1 -> dy(t)/dt/1
  Delay1/1 -> Sum6/1
  "if we went through a \"step\""/1 -> Hold this value/Action
  Hold this value/1(Out1) -> divide by delta T/1
  Sum6/1 -> "if we went through a \"step\""/1, Hold this value/1(In1)
  y(t)/1 -> Sum6/2, Delay1/2, Delay1/1

== system Combined_Experiment_Jan23_2020a/Simulate Plant Dynamics/BLUE Dynamics/BLUE  Dynamics Model ==
  control_inputs : Inport
  Acceleration to Velocity : DiscreteIntegrator  IntegratorMethod=Integration: Backward Euler  SampleTime=-1  ICPrevOutput=DiscIntNeverNeededParam  ICPrevScaledInput=DiscIntNeverNeededParam
  MATLAB Function : MATLAB Function  TreatAsAtomicUnit=on
  Random Number : RandomNumber  Variance=noise_variance_BLUE
  Sum : Sum  Inputs=|++
  Velocity to Position : DiscreteIntegrator  IntegratorMethod=Integration: Backward Euler  InitialCondition=drop_states_BLUE  SampleTime=-1  ICPrevOutput=DiscIntNeverNeededParam  ICPrevScaledInput=DiscIntNeverNeededParam
  states : Outport  VectorParamsAs1DForOutWhenUnconnected=off
  wires:
  control_inputs/1 -> MATLAB Function/1(control_inputs)
  MATLAB Function/1(x_ddot) -> Acceleration to Velocity/1
  Acceleration to Velocity/1 -> Velocity to Position/1
  Velocity to Position/1 -> Sum/1
  Sum/1 -> states/1
  Random Number/1 -> Sum/2

== system Combined_Experiment_Jan23_2020a/Simulate Plant Dynamics/BLUE Dynamics/Sample and Hold Data to Match PhaseSpace (BLUE) ==
  states : Inport
  Constant1 : Constant  Value=serverRate
  Data Store Read2 : DataStoreRead  DataStoreName=Univ_Time
  MATLAB Function : MATLAB Function  TreatAsAtomicUnit=on
  Sample and Hold1 : dspsigops/Sample and Hold  trig=Rising edge  initCond=drop_states_BLUE  latchinput=off
  states_hold : Outport  VectorParamsAs1DForOutWhenUnconnected=off
  wires:
  states/1 -> Sample and Hold1/1
  Data Store Read2/1 -> MATLAB Function/1(TIME)
  Constant1/1 -> MATLAB Function/2(SERVER)
  MATLAB Function/1(y) -> Sample and Hold1/Trigger
  Sample and Hold1/1 -> states_hold/1

== system Combined_Experiment_Jan23_2020a/Simulate Plant Dynamics/BLUE Dynamics/x_dot -> x1 ==
  note: dy/dt ~= (y2-y1)/deltaT
  y(t) : Inport
  Delay1 : Delay  DelayLength=1  InitialConditionSource=Input port
      settings: InputPortMap=u0,p4
  Hold this value : Subsystem  TreatAsAtomicUnit=on
  Sum6 : Sum  Inputs=-+|
  divide by delta T : Gain  Gain=1/baseRate
  "if we went through a \"step\"" : If  IfExpression=u1 ~= 0  ShowElse=off
  dy(t)/dt : Outport  VectorParamsAs1DForOutWhenUnconnected=off
  wires:
  divide by delta T/1 -> dy(t)/dt/1
  Delay1/1 -> Sum6/1
  "if we went through a \"step\""/1 -> Hold this value/Action
  Hold this value/1(Out1) -> divide by delta T/1
  Sum6/1 -> "if we went through a \"step\""/1, Hold this value/1(In1)
  y(t)/1 -> Sum6/2, Delay1/2, Delay1/1

== system Combined_Experiment_Jan23_2020a/Simulate Plant Dynamics/BLUE Dynamics/x_dot -> x2 ==
  note: dy/dt ~= (y2-y1)/deltaT
  y(t) : Inport
  Delay1 : Delay  DelayLength=1  InitialConditionSource=Input port
      settings: InputPortMap=u0,p4
  Hold this value : Subsystem  TreatAsAtomicUnit=on
  Sum6 : Sum  Inputs=-+|
  divide by delta T : Gain  Gain=1/baseRate
  "if we went through a \"step\"" : If  IfExpression=u1 ~= 0  ShowElse=off
  dy(t)/dt : Outport  VectorParamsAs1DForOutWhenUnconnected=off
  wires:
  divide by delta T/1 -> dy(t)/dt/1
  Delay1/1 -> Sum6/1
  "if we went through a \"step\""/1 -> Hold this value/Action
  Hold this value/1(Out1) -> divide by delta T/1
  Sum6/1 -> "if we went through a \"step\""/1, Hold this value/1(In1)
  y(t)/1 -> Sum6/2, Delay1/2, Delay1/1

== system Combined_Experiment_Jan23_2020a/Simulate Plant Dynamics/BLUE Dynamics/x_dot -> x3 ==
  note: dy/dt ~= (y2-y1)/deltaT
  y(t) : Inport
  Delay1 : Delay  DelayLength=1  InitialConditionSource=Input port
      settings: InputPortMap=u0,p4
  Hold this value : Subsystem  TreatAsAtomicUnit=on
  Sum6 : Sum  Inputs=-+|
  divide by delta T : Gain  Gain=1/baseRate
  "if we went through a \"step\"" : If  IfExpression=u1 ~= 0  ShowElse=off
  dy(t)/dt : Outport  VectorParamsAs1DForOutWhenUnconnected=off
  wires:
  divide by delta T/1 -> dy(t)/dt/1
  Delay1/1 -> Sum6/1
  "if we went through a \"step\""/1 -> Hold this value/Action
  Hold this value/1(Out1) -> divide by delta T/1
  Sum6/1 -> "if we went through a \"step\""/1, Hold this value/1(In1)
  y(t)/1 -> Sum6/2, Delay1/2, Delay1/1

== system Combined_Experiment_Jan23_2020a/Simulate Plant Dynamics/BLUE Dynamics/x_dot -> x4 ==
  note: dy/dt ~= (y2-y1)/deltaT
  y(t) : Inport
  Delay1 : Delay  DelayLength=1  InitialConditionSource=Input port
      settings: InputPortMap=u0,p4
  Hold this value : Subsystem  TreatAsAtomicUnit=on
  Sum6 : Sum  Inputs=-+|
  divide by delta T : Gain  Gain=1/baseRate
  "if we went through a \"step\"" : If  IfExpression=u1 ~= 0  ShowElse=off
  dy(t)/dt : Outport  VectorParamsAs1DForOutWhenUnconnected=off
  wires:
  divide by delta T/1 -> dy(t)/dt/1
  Delay1/1 -> Sum6/1
  "if we went through a \"step\""/1 -> Hold this value/Action
  Hold this value/1(Out1) -> divide by delta T/1
  Sum6/1 -> "if we went through a \"step\""/1, Hold this value/1(In1)
  y(t)/1 -> Sum6/2, Delay1/2, Delay1/1

== system Combined_Experiment_Jan23_2020a/Simulate Plant Dynamics/BLUE Dynamics/x_dot -> x7 ==
  note: dy/dt ~= (y2-y1)/deltaT
  y(t) : Inport
  Delay1 : Delay  DelayLength=1  InitialConditionSource=Input port
      settings: InputPortMap=u0,p4
  Hold this value : Subsystem  TreatAsAtomicUnit=on
  Sum6 : Sum  Inputs=-+|
  divide by delta T : Gain  Gain=1/baseRate
  "if we went through a \"step\"" : If  IfExpression=u1 ~= 0  ShowElse=off
  dy(t)/dt : Outport  VectorParamsAs1DForOutWhenUnconnected=off
  wires:
  divide by delta T/1 -> dy(t)/dt/1
  Delay1/1 -> Sum6/1
  "if we went through a \"step\""/1 -> Hold this value/Action
  Hold this value/1(Out1) -> divide by delta T/1
  Sum6/1 -> "if we went through a \"step\""/1, Hold this value/1(In1)
  y(t)/1 -> Sum6/2, Delay1/2, Delay1/1

== system Combined_Experiment_Jan23_2020a/Simulate Plant Dynamics/RED and ARM Dynamics/RED + ARM ==
  Action Port : ActionPort  ActionPortLabel=if(u1 == 4 | u1 == 5 | u1 == 10 | u1 == 11)
  RED + ARM Dynamics : Subsystem

== system Combined_Experiment_Jan23_2020a/Simulate Plant Dynamics/RED and ARM Dynamics/RED Only ==
  Action Port : ActionPort  ActionPortLabel=else
  RED Dynamics : Subsystem

== system Combined_Experiment_Jan23_2020a/From Force//Torque to PWM Signal/Change BLACK Behavior/Calculate Thruster ON//OFF/Rotate Forces to Inertial ==
  "F_b " : Inport
  Rz : Inport  Port=2
  Create Rotation Matrix : MATLAB Function  TreatAsAtomicUnit=on
  Rotate F_b to F_I : Product  Multiplication=Matrix(*)
  F_I : Outport  VectorParamsAs1DForOutWhenUnconnected=off
  wires:
  "F_b "/1 -> Rotate F_b to F_I/2
  Rotate F_b to F_I/1 -> F_I/1
  Create Rotation Matrix/1(C_Ib) -> Rotate F_b to F_I/1
  Rz/1 -> Create Rotation Matrix/1(Rz)

== system Combined_Experiment_Jan23_2020a/From Force//Torque to PWM Signal/Change BLACK Behavior/Calculate Thruster ON//OFF/pseudo-inverse ==
  H : Inport
  Product : Product  Multiplication=Matrix(*)
  Product1 : Product  Inputs=/  Multiplication=Matrix(*)
  Product2 : Product  Multiplication=Matrix(*)
  transpose : PermuteDimensions
  invH : Outport  VectorParamsAs1DForOutWhenUnconnected=off
  wires:
  Product2/1 -> invH/1
  transpose/1 -> Product/2, Product2/1
  Product/1 -> Product1/1
  H/1 -> Product/1, transpose/1
  Product1/1 -> Product2/2

== system Combined_Experiment_Jan23_2020a/From Force//Torque to PWM Signal/Change BLACK Behavior/Calculate Thruster ON//OFF/pseudo-inverse3 ==
  H : Inport
  Product : Product  Multiplication=Matrix(*)
  Product1 : Product  Inputs=/  Multiplication=Matrix(*)
  Product2 : Product  Multiplication=Matrix(*)
  transpose : PermuteDimensions
  invH : Outport  VectorParamsAs1DForOutWhenUnconnected=off
  wires:
  Product2/1 -> invH/1
  transpose/1 -> Product/2, Product2/1
  Product/1 -> Product1/1
  H/1 -> Product/1, transpose/1
  Product1/1 -> Product2/2

== system Combined_Experiment_Jan23_2020a/From Force//Torque to PWM Signal/Change BLUE Behavior/Calculate Thruster ON//OFF/Rotate Forces to Inertial ==
  "F_b " : Inport
  Rz : Inport  Port=2
  Create Rotation Matrix : MATLAB Function  TreatAsAtomicUnit=on
  Rotate F_b to F_I : Product  Multiplication=Matrix(*)
  F_I : Outport  VectorParamsAs1DForOutWhenUnconnected=off
  wires:
  "F_b "/1 -> Rotate F_b to F_I/2
  Rotate F_b to F_I/1 -> F_I/1
  Create Rotation Matrix/1(C_Ib) -> Rotate F_b to F_I/1
  Rz/1 -> Create Rotation Matrix/1(Rz)

== system Combined_Experiment_Jan23_2020a/From Force//Torque to PWM Signal/Change BLUE Behavior/Calculate Thruster ON//OFF/pseudo-inverse ==
  H : Inport
  Product : Product  Multiplication=Matrix(*)
  Product1 : Product  Inputs=/  Multiplication=Matrix(*)
  Product2 : Product  Multiplication=Matrix(*)
  transpose : PermuteDimensions
  invH : Outport  VectorParamsAs1DForOutWhenUnconnected=off
  wires:
  Product2/1 -> invH/1
  transpose/1 -> Product/2, Product2/1
  Product/1 -> Product1/1
  H/1 -> Product/1, transpose/1
  Product1/1 -> Product2/2

== system Combined_Experiment_Jan23_2020a/From Force//Torque to PWM Signal/Change BLUE Behavior/Calculate Thruster ON//OFF/pseudo-inverse2 ==
  H : Inport
  Product : Product  Multiplication=Matrix(*)
  Product1 : Product  Inputs=/  Multiplication=Matrix(*)
  Product2 : Product  Multiplication=Matrix(*)
  transpose : PermuteDimensions
  invH : Outport  VectorParamsAs1DForOutWhenUnconnected=off
  wires:
  Product2/1 -> invH/1
  transpose/1 -> Product/2, Product2/1
  Product/1 -> Product1/1
  H/1 -> Product/1, transpose/1
  Product1/1 -> Product2/2

== system Combined_Experiment_Jan23_2020a/From Force//Torque to PWM Signal/Change RED Behavior/Calculate Thruster ON//OFF/If Action Subsystem ==
  In1 : Inport
  Action Port : ActionPort  ActionPortLabel=if(u1 == 4 | u1 == 5 | u1 == 10 | u1 == 11)
  Out1 : Outport
  wires:
  In1/1 -> Out1/1

== system Combined_Experiment_Jan23_2020a/From Force//Torque to PWM Signal/Change RED Behavior/Calculate Thruster ON//OFF/If Action Subsystem1 ==
  In1 : Inport
  Action Port : ActionPort  ActionPortLabel=else
  Out1 : Outport
  wires:
  In1/1 -> Out1/1

== system Combined_Experiment_Jan23_2020a/From Force//Torque to PWM Signal/Change RED Behavior/Calculate Thruster ON//OFF/If Action Subsystem2 ==
  In1 : Inport
  Action Port : ActionPort  ActionPortLabel=if(u1 == 4 | u1 == 5 | u1 == 10 | u1 == 11)
  Out1 : Outport
  wires:
  In1/1 -> Out1/1

== system Combined_Experiment_Jan23_2020a/From Force//Torque to PWM Signal/Change RED Behavior/Calculate Thruster ON//OFF/If Action Subsystem3 ==
  In1 : Inport
  Action Port : ActionPort  ActionPortLabel=else
  Out1 : Outport
  wires:
  In1/1 -> Out1/1

== system Combined_Experiment_Jan23_2020a/From Force//Torque to PWM Signal/Change RED Behavior/Calculate Thruster ON//OFF/Rotate Forces to Inertial1 ==
  "F_b " : Inport
  Rz : Inport  Port=2
  Create Rotation Matrix : MATLAB Function  TreatAsAtomicUnit=on
  Rotate F_b to F_I : Product  Multiplication=Matrix(*)
  F_I : Outport  VectorParamsAs1DForOutWhenUnconnected=off
  wires:
  "F_b "/1 -> Rotate F_b to F_I/2
  Rotate F_b to F_I/1 -> F_I/1
  Create Rotation Matrix/1(C_Ib) -> Rotate F_b to F_I/1
  Rz/1 -> Create Rotation Matrix/1(Rz)

== system Combined_Experiment_Jan23_2020a/From Force//Torque to PWM Signal/Change RED Behavior/Calculate Thruster ON//OFF/pseudo-inverse1 ==
  H : Inport
  Product : Product  Multiplication=Matrix(*)
  Product1 : Product  Inputs=/  Multiplication=Matrix(*)
  Product2 : Product  Multiplication=Matrix(*)
  transpose : PermuteDimensions
  invH : Outport  VectorParamsAs1DForOutWhenUnconnected=off
  wires:
  Product2/1 -> invH/1
  transpose/1 -> Product/2, Product2/1
  Product/1 -> Product1/1
  H/1 -> Product/1, transpose/1
  Product1/1 -> Product2/2

== system Combined_Experiment_Jan23_2020a/From Force//Torque to PWM Signal/Change RED Behavior/Calculate Thruster ON//OFF/pseudo-inverse2 ==
  H : Inport
  Product : Product  Multiplication=Matrix(*)
  Product1 : Product  Inputs=/  Multiplication=Matrix(*)
  Product2 : Product  Multiplication=Matrix(*)
  transpose : PermuteDimensions
  invH : Outport  VectorParamsAs1DForOutWhenUnconnected=off
  wires:
  Product2/1 -> invH/1
  transpose/1 -> Product/2, Product2/1
  Product/1 -> Product1/1
  H/1 -> Product/1, transpose/1
  Product1/1 -> Product2/2

== system Combined_Experiment_Jan23_2020a/From Torque Command RW/Change RED Behavior/Wheel RPM to PWM/Convert Wheel Rate to Motor Rate ==
  Wheel RPM : Inport
  Divide : Product  Inputs=**
  Gearbox Ratio : Constant  Value=3375/64
  Motor RPM : Outport  VectorParamsAs1DForOutWhenUnconnected=off
  wires:
  Gearbox Ratio/1 -> Divide/2
  Divide/1 -> Motor RPM/1
  Wheel RPM/1 -> Divide/1

== system Combined_Experiment_Jan23_2020a/From Torque Command RW/Change RED Behavior/Wheel RPM to PWM/Delay Bank ==
  Status : Inport
  Delay1 : Delay  DelayLength=1  InitialCondition=0
  Delay2 : Delay  InitialCondition=0
  Delay3 : Delay  DelayLength=4  InitialCondition=0
  Delay4 : Delay  DelayLength=5  InitialCondition=0
  Delay5 : Delay  DelayLength=3  InitialCondition=0
  Mostly zeros? : MinMax  Inputs=6
  StatusVector : Outport  VectorParamsAs1DForOutWhenUnconnected=off
  wires:
  Delay3/1 -> Mostly zeros?/5
  Status/1 -> Delay4/1, Delay3/1, Delay5/1, Delay2/1, Delay1/1, Mostly zeros?/1
  Delay2/1 -> Mostly zeros?/3
  Delay4/1 -> Mostly zeros?/6
  Delay5/1 -> Mostly zeros?/4
  Mostly zeros?/1 -> StatusVector/1
  Delay1/1 -> Mostly zeros?/2

== system Combined_Experiment_Jan23_2020a/From Torque Command RW/Change RED Behavior/Wheel RPM to PWM/Obtain RW Status ==
  GPIO Read1 : embdlinuxlib/GPIO Read  board=Pi 3 Model B  gpio=24  internalResistor=Off  sampleTime=0.1  direction=Input  blockPlatform=Raspberry Pi
      settings: SourceProductBaseCode=SC_BEAGLEBONE_BLUE,RASPPI
  RW_Status : Outport  VectorParamsAs1DForOutWhenUnconnected=off
  wires:
  GPIO Read1/1 -> RW_Status/1

== system Combined_Experiment_Jan23_2020a/From Torque Command RW/Change RED Behavior/Wheel RPM to PWM/Send Direction to Motor Controller ==
  WheelDir : Inport
  GPIO Write : embdlinuxlib/GPIO Write  board=Pi 3 Model B  gpio=21  direction=Output  blockPlatform=Raspberry Pi
      settings: SourceProductBaseCode=SC_BEAGLEBONE_BLUE,RASPPI
  wires:
  WheelDir/1 -> GPIO Write/1

== system Combined_Experiment_Jan23_2020a/From Torque Command RW/Change RED Behavior/Wheel RPM to PWM/Send PWM to Motor Controller ==
  MotorPWM : Inport
  PWM1 : raspberrypiBasiclib/PWM  board=Pi 3 Model B  Pin_=18  Frequency=10  blockPlatform=Raspberry Pi
      settings: SourceProductBaseCode=RASPPI
  wires:
  MotorPWM/1 -> PWM1/1

== system Combined_Experiment_Jan23_2020a/From Torque Command RW/Change RED Behavior/Wheel RPM to PWM/Turn on Motor ==
  EnableSig : Inport
  GPIO Write1 : embdlinuxlib/GPIO Write  board=Pi 3 Model B  gpio=25  direction=Output  blockPlatform=Raspberry Pi
      settings: SourceProductBaseCode=SC_BEAGLEBONE_BLUE,RASPPI
  wires:
  EnableSig/1 -> GPIO Write1/1

== system Combined_Experiment_Jan23_2020a/Grab PhaseSpace Data via UDP/Use Hardware to Obtain States/x_dot -> x1/Hold this value ==
  In1 : Inport
  Action Port : ActionPort  ActionPortLabel=if(u1 ~= 0)
  Out1 : Outport  VectorParamsAs1DForOutWhenUnconnected=off
  wires:
  In1/1 -> Out1/1

== system Combined_Experiment_Jan23_2020a/Grab PhaseSpace Data via UDP/Use Hardware to Obtain States/x_dot -> x10/Hold this value ==
  In1 : Inport
  Action Port : ActionPort  ActionPortLabel=if(u1 ~= 0)
  Out1 : Outport  VectorParamsAs1DForOutWhenUnconnected=off
  wires:
  In1/1 -> Out1/1

== system Combined_Experiment_Jan23_2020a/Grab PhaseSpace Data via UDP/Use Hardware to Obtain States/x_dot -> x11/Hold this value ==
  In1 : Inport
  Action Port : ActionPort  ActionPortLabel=if(u1 ~= 0)
  Out1 : Outport  VectorParamsAs1DForOutWhenUnconnected=off
  wires:
  In1/1 -> Out1/1

== system Combined_Experiment_Jan23_2020a/Grab PhaseSpace Data via UDP/Use Hardware to Obtain States/x_dot -> x12/Hold this value ==
  In1 : Inport
  Action Port : ActionPort  ActionPortLabel=if(u1 ~= 0)
  Out1 : Outport  VectorParamsAs1DForOutWhenUnconnected=off
  wires:
  In1/1 -> Out1/1

== system Combined_Experiment_Jan23_2020a/Grab PhaseSpace Data via UDP/Use Hardware to Obtain States/x_dot -> x16/Hold this value ==
  In1 : Inport
  Action Port : ActionPort  ActionPortLabel=if(u1 ~= 0)
  Out1 : Outport  VectorParamsAs1DForOutWhenUnconnected=off
  wires:
  In1/1 -> Out1/1

== system Combined_Experiment_Jan23_2020a/Grab PhaseSpace Data via UDP/Use Hardware to Obtain States/x_dot -> x17/Hold this value ==
  In1 : Inport
  Action Port : ActionPort  ActionPortLabel=if(u1 ~= 0)
  Out1 : Outport  VectorParamsAs1DForOutWhenUnconnected=off
  wires:
  In1/1 -> Out1/1

== system Combined_Experiment_Jan23_2020a/Grab PhaseSpace Data via UDP/Use Hardware to Obtain States/x_dot -> x18/Hold this value ==
  In1 : Inport
  Action Port : ActionPort  ActionPortLabel=if(u1 ~= 0)
  Out1 : Outport  VectorParamsAs1DForOutWhenUnconnected=off
  wires:
  In1/1 -> Out1/1
